simulink model "Base_isolated_structure_refence"  (R2024a)
settings: Solver=ode4  StartTime=0.0  StopTime=tend  FixedStep=dt  RelTol=1e-3
values from neighbouring files (symbols this model uses):
  alpha0 = 4    [Base_isolated_structure_main.m]
  As = [zeros(24,24) eye(24) zeros(24,6);MK-R*m_RK MC-R*m_RC zeros(24,6);zeros(3,51) eye(3);m_RK m_RC zeros(3,6)]    [Base_isolated_structure_main.m]
  Bs = [zeros(24,6);zeros(24,3) R/m;zeros(3,6);-eye(3) -inv(m)]    [Base_isolated_structure_main.m]
  coe = [A,gamma,beta,n]    [BLWN_training_data_prep.m]    (also in Base_isolated_structure_main.m = [-a_0*dta,dta,b_0-a_0*b_1,b_1,UL]; Inter_story_damped_structure_MFD_main.m = [-a_0*dta,dta,b_0-a_0*b_1,b_1,UL])
  CoeB = [A0,gamma,beta,n]    [Base_isolated_structure_main.m]    (also in Inter_story_damped_structure_MBW_main.m = [A,gamma,beta,n])
  CoeZ = [a,b,k1]    [Base_isolated_structure_main.m]    (also in Inter_story_damped_structure_MBW_main.m)
  Cs = eye(54)    [Base_isolated_structure_main.m]
  Ds = zeros(54,6)    [Base_isolated_structure_main.m]
  dt = 0.002    [BLWN_training_data_prep.m]    (also in Base_isolated_structure_main.m; Inter_story_damped_structure_MBW_main.m; Inter_story_damped_structure_MFD_main.m)
  Fscale = 80    [Base_isolated_structure_main.m]
  GL = zeros(lim-1,1);GL(1)=-alpha    [Base_isolated_structure_main.m]    (also in Inter_story_damped_structure_MFD_main.m)
  k0 = 0.5e-3    (= 0.0005)    [BLWN_training_data_prep.m]    (also in Base_isolated_structure_main.m = 500000; Inter_story_damped_structure_MFD_main.m)
  MBW_locs = All_locs(32:61,2:3)    [Base_isolated_structure_plan.m]
  MBW_N = size(MBW_locs,1)    [Base_isolated_structure_main.m]
  MFD_locs = All_locs(1:31,2:3)    [Base_isolated_structure_plan.m]
  MFD_N = size(MFD_locs,1)    [Base_isolated_structure_main.m]
  Reduce = zeros(6,54);Reduce(:,49:54)=eye(6)    [Base_isolated_structure_main.m]
  UL = i-1    [Base_isolated_structure_main.m]    (also in Inter_story_damped_structure_MFD_main.m)
  uscale = 0.1    [Base_isolated_structure_main.m]
settings Model: Creator=tujia  LastModifiedBy=li292
settings SolverCC: AlgebraicLoopSolver=TrustRegion
settings DataIOCC: ReturnWorkspaceOutputs=off
settings OptimizationCC: LifeSpan=inf
settings DebuggingCC: UnconnectedInputMsg=warning  UnconnectedOutputMsg=warning  UnconnectedLineMsg=warning  ArithmeticOperatorsInVariantConditions=warning
settings ModelReferenceCC: EnableRefExpFcnMdlSchedulingChecks=on
settings SFSimCC: SimUseLocalCustomCode=off  CustomCodeUndefinedFunction=UseInterfaceOnly
settings RTWCC: RTWUseLocalCustomCode=off  GPUComputeCapability=3.5
settings CodeAppCC: StateflowObjectComments=on

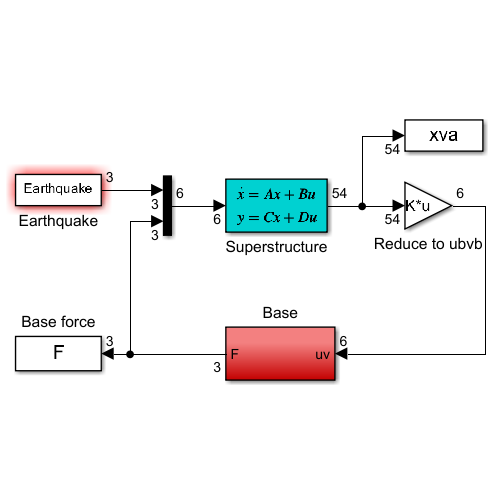
[thumbnail: Simulink's stored preview of the top-level diagram]
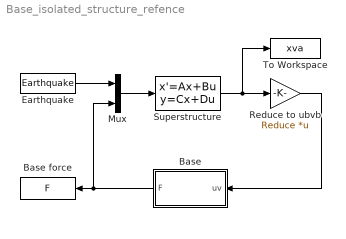
== system Base_isolated_structure_refence ==
  Base : Subsystem
  Base force : ToWorkspace  VariableName=F  SampleTime=dt
      settings: Save2DSignal=2-D array (concatenate along first dimension)
  Earthquake : FromWorkspace  VariableName=Earthquake
  Mux : Mux  Inputs=2
  Reduce to ubvb : Gain  Gain=Reduce  Multiplication=Matrix(K*u)
  Superstructure : StateSpace  A=As  B=Bs  C=Cs  D=Ds  InitialCondition=zeros(54,1)
  To Workspace : ToWorkspace  VariableName=xva  SampleTime=dt
      settings: Save2DSignal=2-D array (concatenate along first dimension)
  wires:
  Reduce to ubvb/1 -> Base/1(uv)
  Mux/1 -> Superstructure/1
  Superstructure/1 -> Reduce to ubvb/1, To Workspace/1
  Earthquake/1 -> Mux/1
  Base/1(F) -> Mux/2, Base force/1

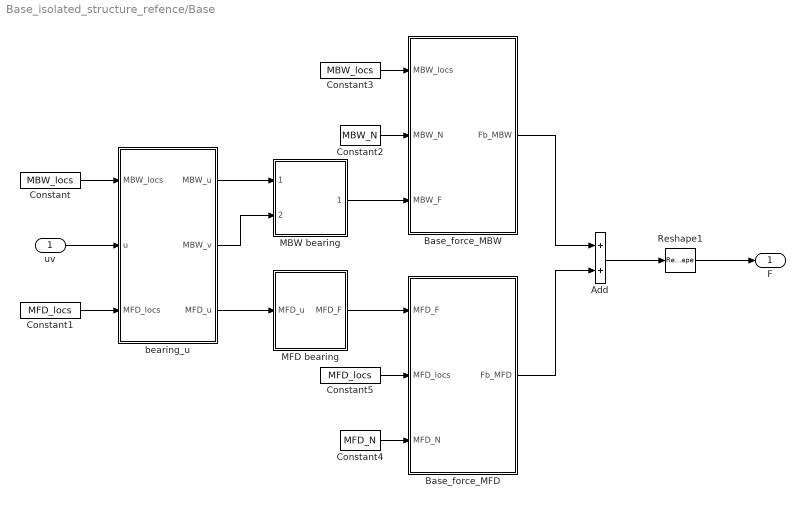
== system Base_isolated_structure_refence/Base ==
  uv : Inport
  Add : Sum
  Base_force_MBW : MATLAB Function  TreatAsAtomicUnit=on
  Base_force_MFD : MATLAB Function  TreatAsAtomicUnit=on
  Constant : Constant  Value=MBW_locs
  Constant1 : Constant  Value=MFD_locs
  Constant2 : Constant  Value=MBW_N
  Constant3 : Constant  Value=MBW_locs
  Constant4 : Constant  Value=MFD_N
  Constant5 : Constant  Value=MFD_locs
  MBW bearing : Subsystem
  MFD bearing : Subsystem
  Reshape1 : Reshape
  bearing_u : MATLAB Function  TreatAsAtomicUnit=on
  F : Outport
  wires:
  Constant/1 -> bearing_u/1(MBW_locs)
  uv/1 -> bearing_u/2(u)
  Constant1/1 -> bearing_u/3(MFD_locs)
  bearing_u/1(MBW_u) -> MBW bearing/1(MBW_u)
  bearing_u/2(MBW_v) -> MBW bearing/2(MBW_v)
  MBW bearing/1(MBW_F) -> Base_force_MBW/3(MBW_F)
  Constant2/1 -> Base_force_MBW/2(MBW_N)
  Constant3/1 -> Base_force_MBW/1(MBW_locs)
  bearing_u/3(MFD_u) -> MFD bearing/1(MFD_u)
  MFD bearing/1(MFD_F) -> Base_force_MFD/1(MFD_F)
  Constant4/1 -> Base_force_MFD/3(MFD_N)
  Constant5/1 -> Base_force_MFD/2(MFD_locs)
  Base_force_MBW/1(Fb_MBW) -> Add/1
  Base_force_MFD/1(Fb_MFD) -> Add/2
  Add/1 -> Reshape1/1
  Reshape1/1 -> F/1

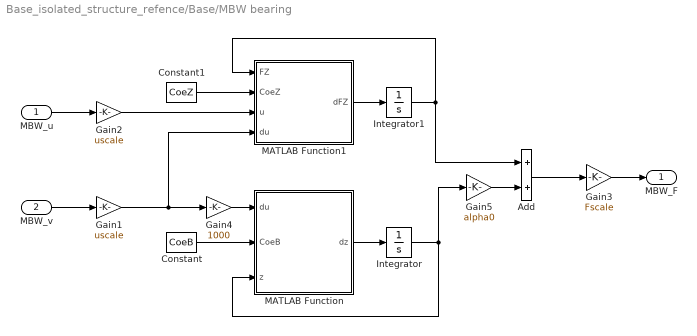
== system Base_isolated_structure_refence/Base/MBW bearing ==
  MBW_u : Inport
  MBW_v : Inport  Port=2
  Add : Sum
  Constant : Constant  Value=CoeB
  Constant1 : Constant  Value=CoeZ
  Gain1 : Gain  Gain=uscale
  Gain2 : Gain  Gain=uscale
  Gain3 : Gain  Gain=Fscale
  Gain4 : Gain  Gain=1000
  Gain5 : Gain  Gain=alpha0
  Integrator : Integrator  InitialCondition=zeros(2*MBW_N,1)
  Integrator1 : Integrator  InitialCondition=zeros(2*MBW_N,1)
  MATLAB Function : MATLAB Function  TreatAsAtomicUnit=on
  MATLAB Function1 : MATLAB Function  TreatAsAtomicUnit=on
  MBW_F : Outport
  wires:
  Constant/1 -> MATLAB Function/2(CoeB)
  MATLAB Function/1(dz) -> Integrator/1
  MBW_u/1 -> Gain2/1
  Constant1/1 -> MATLAB Function1/2(CoeZ)
  MATLAB Function1/1(dFZ) -> Integrator1/1
  MBW_v/1 -> Gain1/1
  Integrator1/1 -> Add/1, MATLAB Function1/1(FZ)
  Add/1 -> Gain3/1
  Gain4/1 -> MATLAB Function/1(du)
  Integrator/1 -> Gain5/1, MATLAB Function/3(z)
  Gain1/1 -> Gain4/1, MATLAB Function1/4(du)
  Gain2/1 -> MATLAB Function1/3(u)
  Gain3/1 -> MBW_F/1
  Gain5/1 -> Add/2

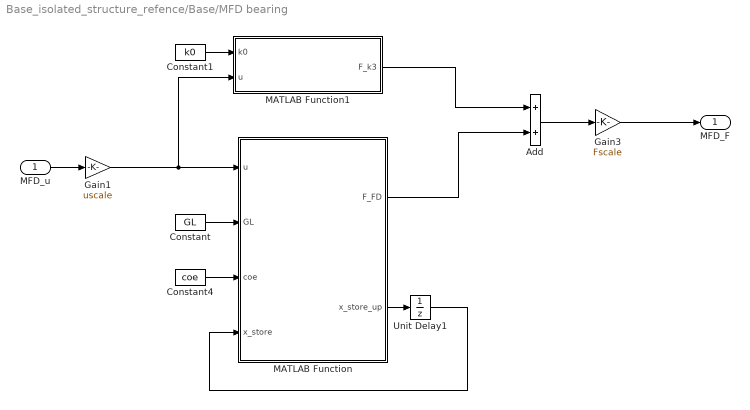
== system Base_isolated_structure_refence/Base/MFD bearing ==
  MFD_u : Inport
  Add : Sum
  Constant : Constant  Value=GL  VectorParams1D=off
  Constant1 : Constant  Value=k0  VectorParams1D=off
  Constant4 : Constant  Value=coe  VectorParams1D=off
  Gain1 : Gain  Gain=uscale
  Gain3 : Gain  Gain=Fscale
  MATLAB Function : MATLAB Function  TreatAsAtomicUnit=on
  MATLAB Function1 : MATLAB Function  TreatAsAtomicUnit=on
  Unit Delay1 : UnitDelay  InitialCondition=[zeros(MFD_N*2,UL)]  SampleTime=-1  HasFrameUpgradeWarning=on
  MFD_F : Outport
  wires:
  Unit Delay1/1 -> MATLAB Function/4(x_store)
  Constant/1 -> MATLAB Function/2(GL)
  MATLAB Function1/1(F_k3) -> Add/1
  Constant1/1 -> MATLAB Function1/1(k0)
  MFD_u/1 -> Gain1/1
  MATLAB Function/2(x_store_up) -> Unit Delay1/1
  Constant4/1 -> MATLAB Function/3(coe)
  Add/1 -> Gain3/1
  MATLAB Function/1(F_FD) -> Add/2
  Gain1/1 -> MATLAB Function1/2(u), MATLAB Function/1(u)
  Gain3/1 -> MFD_F/1

== matlab function Base_isolated_structure_refence/Base/MBW bearing/MATLAB Function ==
  data: du input; dz output; CoeB input; z input
function dz = BoucW(du,CoeB,z)
% coe=[A,gamma,beta,n];
% BoucW=@(du,z)-gamma*abs(du)*abs(z)^(n-1)*z-beta*du*abs(z)^n+A*du;
A=CoeB(1);
gamma=CoeB(2);
beta=CoeB(3);
n=CoeB(4);
dz=-gamma*abs(du).*abs(z).^(n-1).*z-beta*du.*abs(z).^n+A*du;

== matlab function Base_isolated_structure_refence/Base/bearing_u ==
  data: MBW_locs input; u input; MBW_u output; MBW_v output; MFD_locs input; MFD_u output
function [MBW_u,MBW_v,MFD_u] = fcn(MBW_locs,u,MFD_locs)
BW_u1=u(1)-u(3)*MBW_locs(:,2);
BW_u2=u(2)+u(3)*MBW_locs(:,1);
MBW_u = [BW_u1;BW_u2];

BW_v1=u(4)-u(6)*MBW_locs(:,2);
BW_v2=u(5)+u(6)*MBW_locs(:,1);
MBW_v = [BW_v1;BW_v2];

FDZ_u1=u(1)-u(3)*MFD_locs(:,2);
FDZ_u2=u(2)+u(3)*MFD_locs(:,1);
MFD_u = [FDZ_u1;FDZ_u2];

== matlab function Base_isolated_structure_refence/Base/MBW bearing/MATLAB Function1 ==
  data: FZ input; CoeZ input; u input; du input; dFZ output
function dFZ = Zener(FZ,CoeZ,u,du)
% CoeZ=[a,b,k1];
% Zener=@(du,u,f)b*u+k1*du-a*f;
a=CoeZ(1);
b=CoeZ(2);
k1=CoeZ(3);
dFZ=b*u+k1*du-a*FZ;

== matlab function Base_isolated_structure_refence/Base/Base_force_MBW ==
  data: MBW_locs input; MBW_N input; MBW_F input; Fb_MBW output
function Fb_MBW = fcn(MBW_locs,MBW_N,MBW_F)
Fx=sum(MBW_F(1:MBW_N));
Fy=sum(MBW_F(MBW_N+1:end));
Fr=-sum(MBW_F(1:MBW_N).*MBW_locs(:,2))+sum(MBW_F(MBW_N+1:end).*MBW_locs(:,1));
Fb_MBW=[Fx;Fy;Fr];

== matlab function Base_isolated_structure_refence/Base/MFD bearing/MATLAB Function ==
  data: F_FD output; u input; GL input; coe input; x_store input; x_store_up output
function [F_FD,x_store_up] = fcn(u,GL,coe,x_store)
A=coe(1); B=coe(2); C=coe(3); D=coe(4); UL=coe(5);


F_FD = C*x_store(:,1)+D*u;
x_store_up=x_store;
x_store_up(:,2:UL)=x_store(:,1:UL-1);
x_store_up(:,1)=A*x_store(:,1)+B*u-x_store*GL(1:UL);

== matlab function Base_isolated_structure_refence/Base/MFD bearing/MATLAB Function1 ==
  data: k0 input; F_k3 output; u input
function F_k3  = fcn(k0,u)
F_k3=k0*u.^3;

== matlab function Base_isolated_structure_refence/Base/Base_force_MFD ==
  data: MFD_F input; MFD_locs input; MFD_N input; Fb_MFD output
function Fb_MFD = fcn(MFD_F,MFD_locs,MFD_N)
Fx=sum(MFD_F(1:MFD_N));
Fy=sum(MFD_F(MFD_N+1:end));
Fr=-sum(MFD_F(1:MFD_N).*MFD_locs(:,2))+sum(MFD_F(MFD_N+1:end).*MFD_locs(:,1));
Fb_MFD=[Fx;Fy;Fr];
